simulink model "B2B_spv"  (R2017a)
settings: Solver=VariableStepAuto  StartTime=0.0  StopTime=.2  MaxStep=1e-4  RelTol=1e-3
libraries: powerlib x77, powerlib_meascontrol x11, dsparch4 x2
(part 2 of 2)

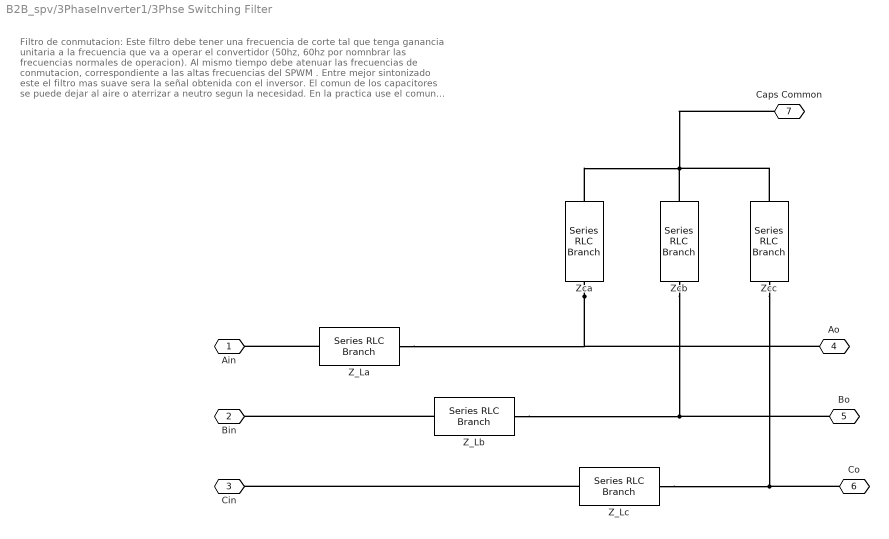
== system B2B_spv/3PhaseInverter1/3Phse Switching Filter ==
  note: Filtro de conmutacion:
      | Este filtro debe tener una frecuencia de corte tal
      | que tenga ganancia unitaria a la frecuencia que va
      | a operar el convertidor (50hz, 60hz por nomnbrar
      | las frecuencias normales de operacion). Al mismo
      | tiempo debe atenuar las frecuencias de conmutacion,
      | correspondiente a las altas frecuencias del SPWM .
      | Entre mejor sintonizado este el filtro mas suave sera
      | la señal obtenida con el inversor. El comun de los
      | capacitores se puede dejar al aire o aterrizar a neutro
      | segun la necesidad. En la practica use el comun al
      | aire para un inversor trifasico de verdad y dio buenos
      | resultados.
  Z_La : powerlib/Elements/Series RLC Branch  LConnTagsString=__new0  RConnTagsString=__new0  BranchType=RL  Resistance=rLf  Inductance=Lf  SetiL0=off  InitialCurrent=0  Capacitance=2.2e-6  Setx0=off  InitialVoltage=0  Measurements=None
  Z_Lb : powerlib/Elements/Series RLC Branch  LConnTagsString=__new0  RConnTagsString=__new0  BranchType=RL  Resistance=rLf  Inductance=Lf  SetiL0=off  InitialCurrent=0  Capacitance=2.2e-6  Setx0=off  InitialVoltage=0  Measurements=None
  Z_Lc : powerlib/Elements/Series RLC Branch  LConnTagsString=__new0  RConnTagsString=__new0  BranchType=RL  Resistance=rLf  Inductance=Lf  SetiL0=off  InitialCurrent=0  Capacitance=2.2e-6  Setx0=off  InitialVoltage=0  Measurements=None
  Zca : powerlib/Elements/Series RLC Branch  LConnTagsString=__new0  RConnTagsString=__new0  BranchType=RC  Resistance=rCf  Inductance=1e-9  SetiL0=off  InitialCurrent=0  Capacitance=Cf  Setx0=off  InitialVoltage=0  Measurements=None
  Zcb : powerlib/Elements/Series RLC Branch  LConnTagsString=__new0  RConnTagsString=__new0  BranchType=RC  Resistance=rCf  Inductance=1e-9  SetiL0=off  InitialCurrent=0  Capacitance=Cf  Setx0=off  InitialVoltage=0  Measurements=None
  Zcc : powerlib/Elements/Series RLC Branch  LConnTagsString=__new0  RConnTagsString=__new0  BranchType=RC  Resistance=rCf  Inductance=1e-9  SetiL0=off  InitialCurrent=0  Capacitance=Cf  Setx0=off  InitialVoltage=0  Measurements=None
  Ain : PMIOPort  Port=1  Side=Left
  Bin : PMIOPort  Port=2  Side=Left
  Cin : PMIOPort  Port=3  Side=Left
  Ao : PMIOPort  Port=4  Side=Right
  Bo : PMIOPort  Port=5  Side=Right
  Co : PMIOPort  Port=6  Side=Right
  Caps Common : PMIOPort  Port=7  Side=Right
  connections:
  Z_Lc/LConn1 -- Cin/RConn1
  Z_Lb/LConn1 -- Bin/RConn1
  Z_La/LConn1 -- Ain/RConn1
  Zca/LConn1 -- Z_La/RConn1 -- Ao/RConn1
  Z_Lc/RConn1 -- Zcc/LConn1 -- Co/RConn1
  Z_Lb/RConn1 -- Zcb/LConn1 -- Bo/RConn1
  Zcb/RConn1 -- Zcc/RConn1 -- Caps Common/RConn1 -- Zca/RConn1

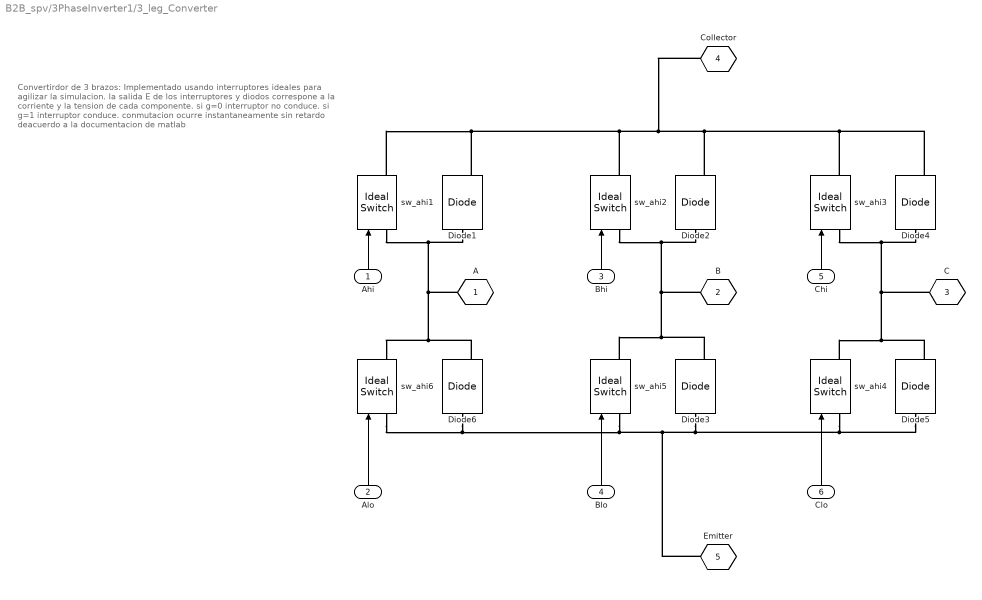
== system B2B_spv/3PhaseInverter1/3_leg_Converter ==
  note: Convertirdor de 3 brazos:
      |
      | Implementado usando interruptores
      | ideales para agilizar la simulacion.
      | la salida E de los interruptores y diodos correspone
      | a la corriente y la tension de cada componente.
      |
      | si g=0 interruptor no conduce.
      | si g=1 interruptor conduce.
      |
      | conmutacion ocurre instantaneamente sin
      | retardo deacuerdo a la documentacion de matlab
  Ahi : Inport
  Alo : Inport  Port=2
  Bhi : Inport  Port=3
  Blo : Inport  Port=4
  Chi : Inport  Port=5
  Clo : Inport  Port=6
   sw_ahi{1..6} (6 alike) : powerlib/Power Electronics/Ideal Switch  Ron=20e-3  Lon=0  IC=0  Rs=1e6  Cs=10e-12  Measurements=on
  Diode{1..6} (6 alike) : powerlib/Power Electronics/Diode  Ron=.2  Lon=0  Vf=0.8  IC=0  UseSnubber=0  Rs=0  Cs=0  Measurements=on
  " A" : PMIOPort  Tag=PMCPort  Port=1  Side=Right
  B : PMIOPort  Tag=PMCPort  Port=2  Side=Right
  C : PMIOPort  Tag=PMCPort  Port=3  Side=Right
  Collector : PMIOPort  Tag=PMCPort  Port=4  Side=Right
  Emitter : PMIOPort  Tag=PMCPort  Port=5  Side=Right
  wires:
  Chi/1 -> " sw_ahi3"/1
  Bhi/1 -> " sw_ahi2"/1
  Blo/1 -> " sw_ahi5"/1
  Ahi/1 -> " sw_ahi1"/1
  Alo/1 -> " sw_ahi6"/1
  Clo/1 -> " sw_ahi4"/1
  connections:
  Diode4/LConn1 -- " sw_ahi3"/LConn1 -- C/RConn1 -- Diode5/RConn1 -- " sw_ahi4"/RConn1
  Diode1/LConn1 -- " sw_ahi1"/LConn1 -- " A"/RConn1 -- Diode6/RConn1 -- " sw_ahi6"/RConn1
  Diode1/RConn1 -- " sw_ahi1"/RConn1 -- " sw_ahi2"/RConn1 -- Collector/RConn1 -- Diode4/RConn1 -- " sw_ahi3"/RConn1 -- Diode2/RConn1
  " sw_ahi6"/LConn1 -- Diode6/LConn1 -- " sw_ahi5"/LConn1 -- Emitter/RConn1 -- Diode5/LConn1 -- " sw_ahi4"/LConn1 -- Diode3/LConn1
  Diode2/LConn1 -- " sw_ahi2"/LConn1 -- B/RConn1 -- " sw_ahi5"/RConn1 -- Diode3/RConn1

== system B2B_spv/3PhaseInverter1/Steper1 ==
  In1 : Inport
  Product : Product
  Step : Step  Time=start_Delay  SampleTime=0
  Out1 : Outport
  wires:
  Product/1 -> Out1/1
  In1/1 -> Product/1
  Step/1 -> Product/2

== system B2B_spv/3PhaseInverter1/Steper2 ==
  In1 : Inport
  Product : Product
  Step : Step  Time=start_Delay  SampleTime=0
  Out1 : Outport
  wires:
  Step/1 -> Product/2
  In1/1 -> Product/1
  Product/1 -> Out1/1

== system B2B_spv/3PhaseInverter1/Steper3 ==
  In1 : Inport
  Product : Product
  Step : Step  Time=start_Delay  SampleTime=0
  Out1 : Outport
  wires:
  Step/1 -> Product/2
  In1/1 -> Product/1
  Product/1 -> Out1/1

== system B2B_spv/3PhaseInverter1/Steper4 ==
  In1 : Inport
  Product : Product
  Step : Step  Time=start_Delay  SampleTime=0
  Out1 : Outport
  wires:
  Product/1 -> Out1/1
  In1/1 -> Product/1
  Step/1 -> Product/2

== system B2B_spv/3PhaseInverter1/Steper5 ==
  In1 : Inport
  Product : Product
  Step : Step  Time=start_Delay  SampleTime=0
  Out1 : Outport
  wires:
  Step/1 -> Product/2
  In1/1 -> Product/1
  Product/1 -> Out1/1

== system B2B_spv/3PhaseInverter1/Steper6 ==
  In1 : Inport
  Product : Product
  Step : Step  Time=start_Delay  SampleTime=0
  Out1 : Outport
  wires:
  Product/1 -> Out1/1
  In1/1 -> Product/1
  Step/1 -> Product/2

== system B2B_spv/Alpha_Beta_PRController/PR Controller_0_ref 1 ==
  ref : Inport
  real : Inport  Port=2
  K1 : Gain  Gain=Kp
  K2 : Gain  Gain=Ki
  Steper6 : Subsystem
  Sum : Sum  Inputs=+-
  Sum1 : Sum  Inputs=+|+
  Transfer Fcn : TransferFcn  Numerator=[1 0]  Denominator=[1 wa (w0)^2]
  Out1 : Outport
  wires:
  Sum1/1 -> Out1/1
  Steper6/1(Out1) -> K2/1, K1/1
  K2/1 -> Transfer Fcn/1
  Transfer Fcn/1 -> Sum1/2
  K1/1 -> Sum1/1
  Sum/1 -> Steper6/1(In1)
  ref/1 -> Sum/1
  real/1 -> Sum/2

== system B2B_spv/Alpha_Beta_PRController/PR Controller_0_ref 3 ==
  ref : Inport
  real : Inport  Port=2
  K1 : Gain  Gain=Kp
  K2 : Gain  Gain=Ki
  Steper6 : Subsystem
  Sum : Sum  Inputs=+-
  Sum1 : Sum  Inputs=+|+
  Transfer Fcn : TransferFcn  Numerator=[1 0]  Denominator=[1 wa (w0)^2]
  Out1 : Outport
  wires:
  real/1 -> Sum/2
  ref/1 -> Sum/1
  Sum/1 -> Steper6/1(In1)
  K1/1 -> Sum1/1
  Transfer Fcn/1 -> Sum1/2
  K2/1 -> Transfer Fcn/1
  Steper6/1(Out1) -> K1/1, K2/1
  Sum1/1 -> Out1/1

== system B2B_spv/PowerControlLoop_4CSI/Alpha_Beta_PRController ==
  note: Lazo de control Resonante para la
      | corriente trifasica en variables alpha beta.
  Ia_ref : Inport
  ib_ref : Inport  Port=2
  I3 : Inport  Port=3
  Alpha-Beta-Zero to abc : powerlib_meascontrol/Transformations/Alpha-Beta-Zero to abc
      settings: SourceProductName=Simscape Power Systems  SourceProductBaseCode=PS
  Demux : Demux  Outputs=3
  Mux1 : Mux  Inputs=3
  PR Controller_0_ref 1 : Subsystem
      mask Display:
      | port_label('input',1,'ref')
      | port_label('input',2,'sens')
      | port_label('output',1,'out')
      | 
      | plot(.4+[0:.01:pi/10], .32+sin(40*[0:.01:pi/10])/13)
      | 
      | plot([.4 .6],.05+[.5 .7])
      | plot([.4 .6],.05+[.9 .7])
      | plot([.4 .4],.05+[.9 .5])
      | 
      | text(.27,.37,'\fontsize{25} \int', 'texmode', 'on')
  PR Controller_0_ref 3 : Subsystem
      mask Display:
      | port_label('input',1,'ref')
      | port_label('input',2,'sens')
      | port_label('output',1,'out')
      | 
      | plot(.4+[0:.01:pi/10], .32+sin(40*[0:.01:pi/10])/13)
      | 
      | plot([.4 .6],.05+[.5 .7])
      | plot([.4 .6],.05+[.9 .7])
      | plot([.4 .4],.05+[.9 .5])
      | 
      | text(.27,.37,'\fontsize{25} \int', 'texmode', 'on')
  abc to Alpha-Beta-Zero : powerlib_meascontrol/Transformations/abc to Alpha-Beta-Zero
      settings: SourceProductName=Simscape Power Systems
  Iab_act : Outport
  wires:
  I3/1 -> abc to Alpha-Beta-Zero/1
  Demux/2 -> PR Controller_0_ref 1/2(real)
  PR Controller_0_ref 1/1(Out1) -> Mux1/2
  Mux1/1 -> Alpha-Beta-Zero to abc/1
  Alpha-Beta-Zero to abc/1 -> Iab_act/1
  abc to Alpha-Beta-Zero/1 -> Demux/1
  ib_ref/1 -> PR Controller_0_ref 1/1(ref)
  Ia_ref/1 -> PR Controller_0_ref 3/1(ref)
  PR Controller_0_ref 3/1(Out1) -> Mux1/1
  Demux/3 -> Mux1/3
  Demux/1 -> PR Controller_0_ref 3/2(real)

== system B2B_spv/Alpha_Beta_PRController/PR Controller_0_ref 1/Steper6 ==
  In1 : Inport
  Product : Product
  Step : Step  Time=start_delay  SampleTime=0
  Out1 : Outport
  wires:
  Step/1 -> Product/2
  In1/1 -> Product/1
  Product/1 -> Out1/1

== system B2B_spv/Alpha_Beta_PRController/PR Controller_0_ref 3/Steper6 ==
  In1 : Inport
  Product : Product
  Step : Step  Time=start_delay  SampleTime=0
  Out1 : Outport
  wires:
  Product/1 -> Out1/1
  In1/1 -> Product/1
  Step/1 -> Product/2

== system B2B_spv/PowerControlLoop_4CSI/Alpha_Beta_PRController/PR Controller_0_ref 1 ==
  ref : Inport
  real : Inport  Port=2
  K1 : Gain  Gain=Kp
  K2 : Gain  Gain=Ki
  Steper6 : Subsystem
  Sum : Sum  Inputs=+-
  Sum1 : Sum  Inputs=+|+
  Transfer Fcn : TransferFcn  Numerator=[1 0]  Denominator=[1 wa (w0)^2]
  Out1 : Outport
  wires:
  Sum1/1 -> Out1/1
  Steper6/1(Out1) -> K2/1, K1/1
  K2/1 -> Transfer Fcn/1
  Transfer Fcn/1 -> Sum1/2
  K1/1 -> Sum1/1
  Sum/1 -> Steper6/1(In1)
  ref/1 -> Sum/1
  real/1 -> Sum/2

== system B2B_spv/PowerControlLoop_4CSI/Alpha_Beta_PRController/PR Controller_0_ref 3 ==
  ref : Inport
  real : Inport  Port=2
  K1 : Gain  Gain=Kp
  K2 : Gain  Gain=Ki
  Steper6 : Subsystem
  Sum : Sum  Inputs=+-
  Sum1 : Sum  Inputs=+|+
  Transfer Fcn : TransferFcn  Numerator=[1 0]  Denominator=[1 wa (w0)^2]
  Out1 : Outport
  wires:
  real/1 -> Sum/2
  ref/1 -> Sum/1
  Sum/1 -> Steper6/1(In1)
  K1/1 -> Sum1/1
  Transfer Fcn/1 -> Sum1/2
  K2/1 -> Transfer Fcn/1
  Steper6/1(Out1) -> K1/1, K2/1
  Sum1/1 -> Out1/1

== system B2B_spv/PowerControlLoop_4CSI/Alpha_Beta_PRController/PR Controller_0_ref 1/Steper6 ==
  In1 : Inport
  Product : Product
  Step : Step  Time=start_delay  SampleTime=0
  Out1 : Outport
  wires:
  Step/1 -> Product/2
  In1/1 -> Product/1
  Product/1 -> Out1/1

== system B2B_spv/PowerControlLoop_4CSI/Alpha_Beta_PRController/PR Controller_0_ref 3/Steper6 ==
  In1 : Inport
  Product : Product
  Step : Step  Time=start_delay  SampleTime=0
  Out1 : Outport
  wires:
  Product/1 -> Out1/1
  In1/1 -> Product/1
  Step/1 -> Product/2

== matlab function B2B_spv/3PhaseInverter/not_pwm1 ==
  data: u input; y output
function y = fcn(u)
%#codegen

if(u==0 || u<0)
    a=5;
else
    a=0;
end;

y = a;

== matlab function B2B_spv/3PhaseInverter/not_pwm ==
  data: u input; y output
function y = fcn(u)
%#codegen

if(u==0 || u<0)
    a=15;
else
    a=0;
end;

y = a;

== matlab function B2B_spv/3PhaseInverter/not_pwm2 ==
  data: u input; y output
function y = fcn(u)
%#codegen

if(u==0 || u<0)
    a=5;
else
    a=0;
end;

y = a;

== matlab function B2B_spv/3PhaseInverter1/not_pwm ==
  data: u input; y output
function y = fcn(u)
%#codegen

if(u==0 || u<0)
    a=15;
else
    a=0;
end;

y = a;

== matlab function B2B_spv/3PhaseInverter1/not_pwm1 ==
  data: u input; y output
function y = fcn(u)
%#codegen

if(u==0 || u<0)
    a=5;
else
    a=0;
end;

y = a;

== matlab function B2B_spv/3PhaseInverter1/not_pwm2 ==
  data: u input; y output
function y = fcn(u)
%#codegen

if(u==0 || u<0)
    a=5;
else
    a=0;
end;

y = a;

== matlab function B2B_spv/PowerControlLoop_4CSI/Instantaneous p-q transformation ==
  data: va input; p output; vb input; vc input; ia input; ib input; ic input; q output; p0 output; iac output; ibc output; icc output; ialphC output; ibetaC output; ValA output; VbetA output
function [p, q, p0, iac, ibc, icc, ialphC, ibetaC, ValA, VbetA] = fcn(va, vb, vc, ia, ib, ic)
% Esta funcion calcula la potencia activa y reactiva instantanea
% dados 3 tensiones y 3 corrientes instantaneas.
% para esto se usa version de la transformada de clarke cuya potencia es 
% invariante (power invariant clarke transform).


pi_clarke = [[1 -1/2 -1/2]; [0 sqrt(3)/2 -sqrt(3)/2]; [1/sqrt(2) 1/sqrt(2) 1/sqrt(2)]]*sqrt(2/3);%matriz de clarke

tv = pi_clarke*[va;vb;vc];% transformada de las tensiones
ti = pi_clarke*[ia;ib;ic];%trasnformada de las corrientes

valph = tv(1);% se separa los valores de las transformadas de tension
vbet = tv(2);
v0 = tv(3);

ValA = valph;
VbetA = vbet;

ialph = ti(1);% se separa los valores de la transformda de corriente
ibet = ti(2);
i0 = ti(3);

paux=valph*ialph+vbet*ibet;
if(paux > 20e4)
    paux=20e4;
end;
if(paux < -20e4)
    paux = -20e-4;
end;

p = paux; % potencia activa instantanea

qaux=vbet*ialph-valph*ibet;

if(qaux>20e4)
    qaux=20e4;
end;
if(qaux<-20e4)
    qaux=-20e4;
end;
q = qaux; % potencia reactiva instantanea


p0 = v0*i0; % potencia instantanea de secuencia 0.



mat2cur = [valph vbet; vbet valph]; % matriz para pasar de potencia
% a corrientes por medio de una matriz de tensiones en alpha beta.

det = 1/(valph^2+vbet^2); % constante auxiliar
if(abs(det)<=100*eps(0))
    det=10*eps(0);
end;

mat2cur = mat2cur*det; % matriz final para pasar a corrientes



IabetC = mat2cur*[0; -q]; % vector corriente de compensacion en alpha beta

%inv_clarke = inv([[1 -1/2 -1/2]; [0 sqrt(3)/2 -sqrt(3)/2]; [1/sqrt(2) 1/sqrt(2) 1/sqrt(2)]]*sqrt(2/3));%matriz de clarke

ialphCaux = IabetC(1);
ibetaCaux = IabetC(2);

ilim=10e3;

if(ialphCaux>ilim)
    ialphCaux=ilim;
end;
if(ialphCaux<-ilim)
    ialphCaux =-ilim;    
end;
if(isnan(ialphCaux))
    ialphCaux=0;
end;
%---------------------
if(ibetaCaux>ilim)
    ibetaCaux=ilim;
end;
if(ibetaCaux<-ilim)
    ibetaCaux=-ilim;    
end;
if(isnan(ibetaCaux))
    ibetaCaux=0;
end;
ialphC = ialphCaux;
ibetaC = ibetaCaux;


Icom = pi_clarke\[IabetC(1); IabetC(2); 0];

iacaux = Icom(1);
ibcaux = Icom(2);
iccaux = Icom(3);

if(iacaux>ilim)
    iacaux=ilim;
end;
if(iacaux<-ilim)
    iacaux =-ilim;    
end;
if(isnan(iacaux))
    iacaux=0;
end;
%---------------------
if(ibcaux>ilim)
    ibcaux=ilim;
end;
if(ibcaux<-ilim)
    ibcaux =-ilim;    
end;

if(isnan(ibcaux))
    ibcaux=0;
end;
%-------------
if(iccaux>ilim)
    iccaux=ilim;
end;
if(iccaux<-ilim)
    iccaux =-ilim;    
end;

if(isnan(iccaux))
    iccaux=0;
end;
%-----------------
iac = iacaux;
ibc = ibcaux;
icc = iccaux;

== matlab function B2B_spv/PowerControlLoop_4CSI/PQ2AlphBetaCurrents ==
  data: Va input; Ia output; Vb input; p input; q input; Ib output
function [Ia, Ib] = fcn(Va, Vb, p, q)
%#codegen

% divide by zero protection
if(abs((Va^2+Vb^2))<=1000*eps(0))
    det = 1/eps(0);
else
    det = 1/(Va^2+Vb^2); % constante auxiliar
end;
%det = 1/(Va^2+Vb^2);

Mat = det*[Va Vb; Vb -Va];
Iab = Mat*[p;q];

Iaaux = Iab(1);
Ibaux = Iab(2);

ilim=1e3;

if(Iaaux>ilim)
    Iaaux=ilim;
end;
if(Iaaux<-ilim)
    Iaaux =-ilim;    
end;

if(isnan(Iaaux))
    Iaaux=0;
end;
%-----------------


if(Ibaux>ilim)
    Ibaux=ilim;
end;
if(Ibaux<-ilim)
    Ibaux =-ilim;    
end;

if(isnan(Ibaux))
    Ibaux=0;
end;
%-----------------


Ia = Iaaux;
Ib = Ibaux;
